simulink model "collision"  (R2018a)
settings: Solver=FixedStepDiscrete  StartTime=0.0  StopTime=10  FixedStep=0.1  RelTol=1e-3  EnableMultiTasking=on
settings Model: Creator=Vadson  LastModifiedBy=Carapinha
settings SolverCC: AutoInsertRateTranBlk=on
settings DataIOCC: LimitDataPoints=on
settings OptimizationCC: LifeSpan=inf
settings DebuggingCC: AllowSymbolicDim=off  SFUnexpectedBacktrackingDiag=warning  SFNoUnconditionalDefaultTransitionDiag=warning  SFExecutionAtInitializationDiag=none
settings CodeAppCC: StateflowObjectComments=on
settings GRTTargetCC: TargetLangStandard=C89/C90 (ANSI)  GeneratePreprocessorConditionals=Disable all
settings ConfigComp: CovMetricSettings=dw  CovHtmlReporting=on  CovSaveCumulativeToWorkspaceVar=on  CovSaveSingleToWorkspaceVar=on  CovShowResultsExplorer=off  CovExternalEMLEnable=off  CovSFcnEnable=off

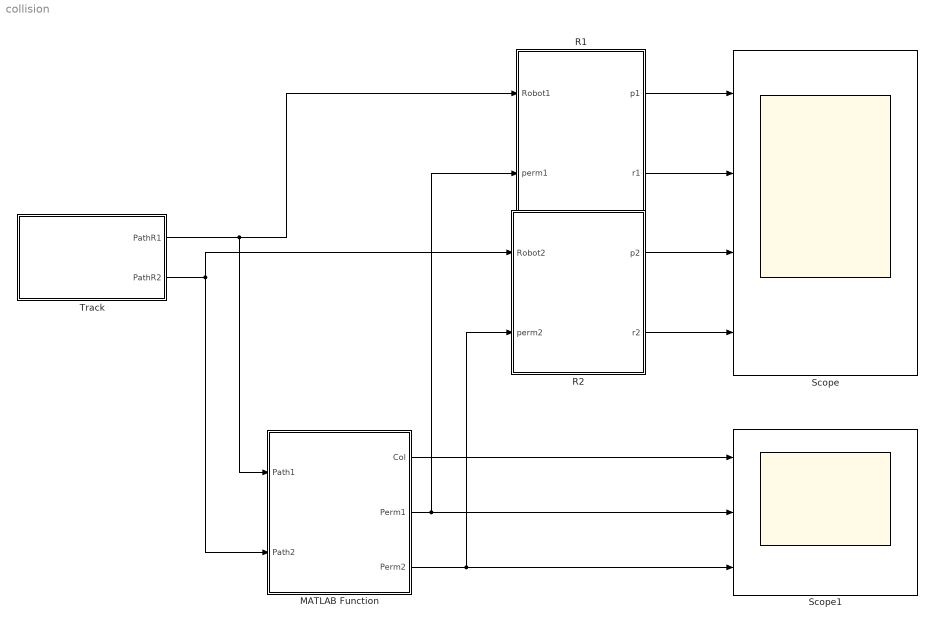
== system collision ==
  MATLAB Function : MATLAB Function  TreatAsAtomicUnit=on
  R1 : Stateflow chart  TreatAsAtomicUnit=on
  R2 : Stateflow chart  TreatAsAtomicUnit=on
  Scope : Scope  NumInputPorts=4
  Scope1 : Scope  NumInputPorts=3
  Track : MATLAB Function  TreatAsAtomicUnit=on
  wires:
  Track/2(PathR2) -> R2/1(Robot2), MATLAB Function/2(Path2)
  R1/1(p1) -> Scope/1
  Track/1(PathR1) -> R1/1(Robot1), MATLAB Function/1(Path1)
  MATLAB Function/2(Perm1) -> Scope1/2, R1/2(perm1)
  MATLAB Function/3(Perm2) -> Scope1/3, R2/2(perm2)
  MATLAB Function/1(Col) -> Scope1/1
  R1/2(r1) -> Scope/2
  R2/1(p2) -> Scope/3
  R2/2(r2) -> Scope/4

== stateflow chart collision/R2 ==
  state s0
    p2 = 0;
    r2 = Robot2(1);
  state s1
    p2 = 1;
    r2 = Robot2(2);
  state s2
    p2 = 2;
    r2 = Robot2(3);
  state s3
    p2 = 3;
    r2 = Robot2(4);
  state s4
    p2 = 4;
    r2 = Robot2(5);
  state s5
    p2=5;
    r2 = Robot2(6);
  (default) -> s0
  s0 -> s1 : [perm2 == 1]
  s1 -> s2 : [perm2 == 1]
  s2 -> s3 : [perm2 == 1]
  s3 -> s4 : [perm2 == 1]
  s4 -> s5 : [perm2 == 1]
  data: p2 output; Robot2 input; perm2 input; r2 output

== matlab function collision/Track ==
  data: PathR1 output; PathR2 output
function [PathR1, PathR2] = Track()

PathR1 = zeros(1,6);
PathR2 = zeros(1,6);

for k = 1:6
   PathR1(1,k) = randi(10,1);
   PathR2(1,k) = randi(10,1);
end

== stateflow chart collision/R1 ==
  state State0
    p1 = 0;
    r1 = Robot1(1);
  state State1
    p1 = 1;
    r1 = Robot1(2);
  state State2
    p1 = 2;
    r1 = Robot1(3);
  state State3
    p1=3;
    r1 = Robot1(4);
  state State4
    p1=4;
    r1 = Robot1(5);
  state State5
    p1=5;
    r1 = Robot1(6);
  (default) -> State0
  State0 -> State1 : [perm1 == 1]
  State1 -> State2 : [perm1 == 1]
  State2 -> State3 : [perm1 == 1]
  State3 -> State4 : [perm1 == 1]
  State4 -> State5 : [perm1 == 1]
  data: p1 output; Robot1 input; perm1 input; r1 output

== matlab function collision/MATLAB Function ==
  data: Path1 input; Col output; Path2 input; Perm1 output; Perm2 output
function [Col, Perm1 , Perm2] = Control(Path1, Path2)

for i = 1:length(Path1)
    if(Path1(i) == Path2(i))
        Col = 1;
        Perm1 = 1;
        Perm2 = 0;
    else 
        Col = 0;
        Perm1 = 1;
        Perm2 = 1;        
    end
end
